simulink model "RelOrbSim"  (R2021b)
settings: Solver=ode3  StartTime=0.0  StopTime=300  FixedStep=0.1  MaxStep=0.1  RelTol=1e-13  AbsTol=1e-16
values from neighbouring files (symbols this model uses):
  cHorizon = 12    [MAIN.m]
  Controller_Engaged_flag = 1    [MAIN.m]
  CostA = 10    [MAIN.m]
  CostB = 10    [MAIN.m]
  CostRelG = 1e4    (= 10000)    [MAIN.m]
  ctrl_flag = 1    [MAIN.m]
  g0 = 9.81    [MAIN.m]
  Isp = 250    [MAIN.m]
  J2_flag = 1    [MAIN.m]
  LinSysMat = zeros(6,6)    [MAIN.m]
  M0 = M0_next    [MAIN.m]
  pHorizon = 60    [MAIN.m]
  RangeLims = [76 75.8]    [MAIN.m]
  Tmax = 0.001    [MAIN.m]
  Ts_MPC = 5    [MAIN.m]
  Y0_Chaser = Y0_Chaser_next    [MAIN.m]
  Y0_Target = Y0_Target_next    [MAIN.m]
settings Model: SimulationMode=accelerator  Creator=vvh19  LastModifiedBy=vvh19
settings SolverCC: ZeroCrossAlgorithm=Adaptive
settings DebuggingCC: IgnoredZcDiagnostic=none

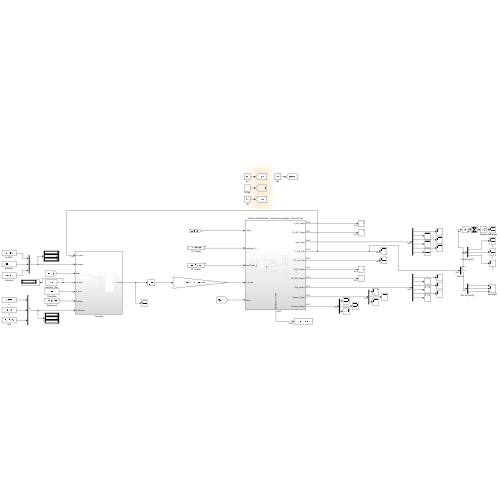
[thumbnail: Simulink's stored preview of the top-level diagram]
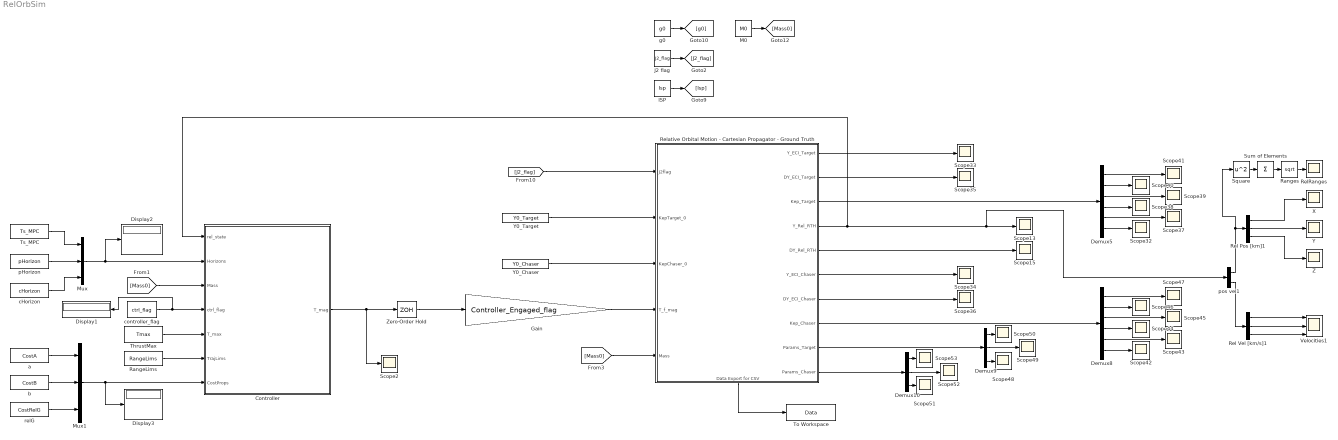
== system RelOrbSim ==
  Controller : Subsystem
  Demux10 : Demux  Outputs=3
  Demux5 : Demux  Outputs=6
  Demux8 : Demux  Outputs=6
  Demux9 : Demux  Outputs=3
  Display1 : Display
  Display2 : Display
  Display3 : Display
  Gain : Gain  Gain=Controller_Engaged_flag
  ISP : Constant  Value=Isp
  J2 flag : Constant  Value=J2_flag
  M0 : Constant  Value=M0
  Mux : Mux  Inputs=3
  Mux1 : Mux  Inputs=3
  RangeLims : Constant  Value=RangeLims
  Ranges : Sqrt  SaturateOnIntegerOverflow=on
  Rel Pos [km]1 : Demux  Outputs=3
  Rel Vel [km/s]1 : Demux  Outputs=3
  RelRanges : Scope
  Relative Orbital Motion - Cartesian Propagator - Ground Truth : Subsystem
      settings: PortSchema="{\"entries\":[{\"content\":{\"sides\":[{\"content\":{\"connectorIds\":[\"In1\",\"In2\",\"In3\",\"In4\",\"In5\"]},\"type\":\"ConnectorPlacement.EquallySpacedRectSide\",\"uuid\":\"460fd9d6-cd5d-4b76-b443-bcd8299910b0\"},{\"content\":{\"connectorIds\":[\"Out1\",\"Out2\",\"Out3\",\"Out4\",\"Out5\",\"Out6\",\"Out7\",\"Out8\",\"Out9\",\"Out10\"],\"side\":\"RIGHT\"},\"type\":\"ConnectorPlacement.EquallySpacedRectSide\",\"uuid\":\"3d6e3c75-f9f1-4d35-a2af-329ac414795a\"},{\"content\":{\"connectorIds\":[],\"side\":\"TOP\"},\"type\":\"ConnectorPlacement.EquallySpacedRectSide\",\"uuid\":\"ebced619-41c7-4fff-b50c-f89432cfa79e\"},{\"content\":{\"connectorIds\":[\"Out11\"],\"side\":\"BOTTOM\"},\"type\":\"ConnectorPlacement.EquallySpacedRectSide\",\"uuid\":\"f646bff0-d8f7-4748-8894-8aba1f3e2913\"}]},\"type\":\"ConnectorPlacement.EquallySpacedConnector\",\"uuid\":\"aa7fbb89-a653-4056-80bd-de050f54cf23\"}],\"packageUris\":[\"http://schema.mathworks.com/mf0/Connector/R2020b\"],\"version\":\"1.0\"}"
  Scope{2,13,15,32..53} (25 alike) : Scope
  Square : Math  Operator=square  SaturateOnIntegerOverflow=on
  Sum of Elements : Sum  Inputs=+
  ThrustMax : Constant  Value=Tmax
  To Workspace : ToWorkspace  VariableName=Data  SampleTime=-1
      settings: Save2DSignal=2-D array (concatenate along first dimension)
  Ts_MPC : Constant  Value=Ts_MPC
  Velocities1 : Scope  NumInputPorts=3
  X : Scope
  Y : Scope
  Y0_Chaser : Constant  Value=Y0_Chaser
  Y0_Target : Constant  Value=Y0_Target
  Z : Scope
  Zero-Order Hold : ZeroOrderHold  SampleTime=Ts_MPC
  a : Constant  Value=CostA
  b : Constant  Value=CostB
  cHorizon : Constant  Value=cHorizon
  controller_flag : Constant  Value=ctrl_flag
  g0 : Constant  Value=g0
  pHorizon : Constant  Value=pHorizon
  pos vel1 : Demux  Outputs=2
  relG : Constant  Value=CostRelG
  wires:
  ISP/1 -> [Isp]
  J2 flag/1 -> [J2_flag]
  M0/1 -> [Mass0]
  g0/1 -> [g0]
  Y0_Target/1 -> Relative Orbital Motion - Cartesian Propagator - Ground Truth/2(KepTarget_0)
  Y0_Chaser/1 -> Relative Orbital Motion - Cartesian Propagator - Ground Truth/3(KepChaser_0)
  [J2_flag] -> Relative Orbital Motion - Cartesian Propagator - Ground Truth/1(J2flag)
  Relative Orbital Motion - Cartesian Propagator - Ground Truth/4(Y_Rel_RTH) -> Scope13/1, pos vel1/1, Controller/1(rel_state)
  Relative Orbital Motion - Cartesian Propagator - Ground Truth/5(DY_Rel_RTH) -> Scope15/1
  Relative Orbital Motion - Cartesian Propagator - Ground Truth/1(Y_ECI_Target) -> Scope33/1
  Relative Orbital Motion - Cartesian Propagator - Ground Truth/6(Y_ECI_Chaser) -> Scope34/1
  Relative Orbital Motion - Cartesian Propagator - Ground Truth/2(DY_ECI_Target) -> Scope35/1
  Relative Orbital Motion - Cartesian Propagator - Ground Truth/7(DY_ECI_Chaser) -> Scope36/1
  Demux5/3 -> Scope39/1
  Demux5/2 -> Scope40/1
  Relative Orbital Motion - Cartesian Propagator - Ground Truth/3(Kep_Target) -> Demux5/1
  Demux5/4 -> Scope38/1
  Demux5/6 -> Scope32/1
  Demux5/1 -> Scope41/1
  Demux5/5 -> Scope37/1
  Demux8/5 -> Scope43/1
  Demux8/1 -> Scope47/1
  Demux8/6 -> Scope42/1
  Demux8/4 -> Scope44/1
  Relative Orbital Motion - Cartesian Propagator - Ground Truth/8(Kep_Chaser) -> Demux8/1
  Demux8/2 -> Scope46/1
  Demux8/3 -> Scope45/1
  Relative Orbital Motion - Cartesian Propagator - Ground Truth/11(Data Export for CSV) -> To Workspace/1
  Demux9/2 -> Scope49/1
  Demux9/3 -> Scope48/1
  Demux9/1 -> Scope50/1
  Relative Orbital Motion - Cartesian Propagator - Ground Truth/9(Params_Target) -> Demux9/1
  Demux10/1 -> Scope53/1
  Demux10/3 -> Scope51/1
  Demux10/2 -> Scope52/1
  Relative Orbital Motion - Cartesian Propagator - Ground Truth/10(Params_Chaser) -> Demux10/1
  pos vel1/1 -> Square/1, Rel Pos [km]1/1
  Rel Pos [km]1/1 -> X/1
  Rel Pos [km]1/3 -> Z/1
  pos vel1/2 -> Rel Vel [km/s]1/1
  Rel Pos [km]1/2 -> Y/1
  Rel Vel [km/s]1/1 -> Velocities1/1
  Rel Vel [km/s]1/2 -> Velocities1/2
  Rel Vel [km/s]1/3 -> Velocities1/3
  controller_flag/1 -> Display1/1, Controller/4(ctrl_flag)
  Square/1 -> Sum of Elements/1
  Sum of Elements/1 -> Ranges/1
  Ranges/1 -> RelRanges/1
  [Mass0] -> Controller/3(Mass)
  [Mass0] -> Relative Orbital Motion - Cartesian Propagator - Ground Truth/5(Mass)
  ThrustMax/1 -> Controller/5(T_max)
  Mux/1 -> Controller/2(Horizons), Display2/1
  pHorizon/1 -> Mux/2
  cHorizon/1 -> Mux/3
  Ts_MPC/1 -> Mux/1
  RangeLims/1 -> Controller/6(TrajLims)
  Mux1/1 -> Controller/7(CostProps), Display3/1
  a/1 -> Mux1/1
  b/1 -> Mux1/2
  Gain/1 -> Relative Orbital Motion - Cartesian Propagator - Ground Truth/4(T_f_mag)
  Controller/1(T_mag) -> Zero-Order Hold/1, Scope2/1
  Zero-Order Hold/1 -> Gain/1
  relG/1 -> Mux1/3

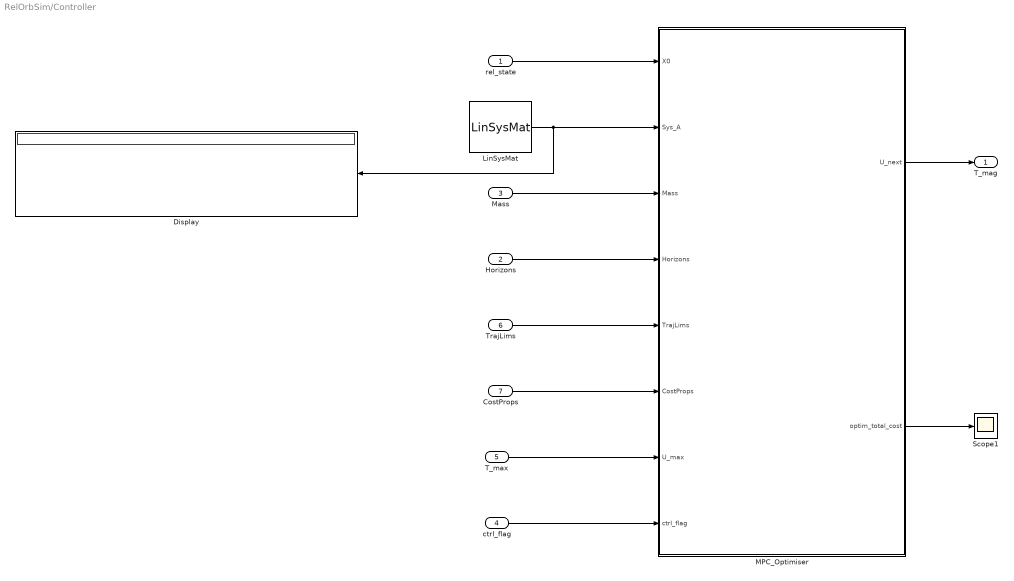
== system RelOrbSim/Controller ==
  rel_state : Inport
  Horizons : Inport  Port=2
  Mass : Inport  Port=3
  ctrl_flag : Inport  Port=4
  T_max : Inport  Port=5
  TrajLims : Inport  Port=6
  CostProps : Inport  Port=7
  Display : Display
  LinSysMat : Constant  Value=LinSysMat
  MPC_Optimiser : MATLAB Function  TreatAsAtomicUnit=on
  Scope1 : Scope
  T_mag : Outport
  wires:
  LinSysMat/1 -> Display/1, MPC_Optimiser/2(Sys_A)
  rel_state/1 -> MPC_Optimiser/1(X0)
  Mass/1 -> MPC_Optimiser/3(Mass)
  T_max/1 -> MPC_Optimiser/7(U_max)
  MPC_Optimiser/2(optim_total_cost) -> Scope1/1
  MPC_Optimiser/1(U_next) -> T_mag/1
  ctrl_flag/1 -> MPC_Optimiser/8(ctrl_flag)
  TrajLims/1 -> MPC_Optimiser/5(TrajLims)
  Horizons/1 -> MPC_Optimiser/4(Horizons)
  CostProps/1 -> MPC_Optimiser/6(CostProps)

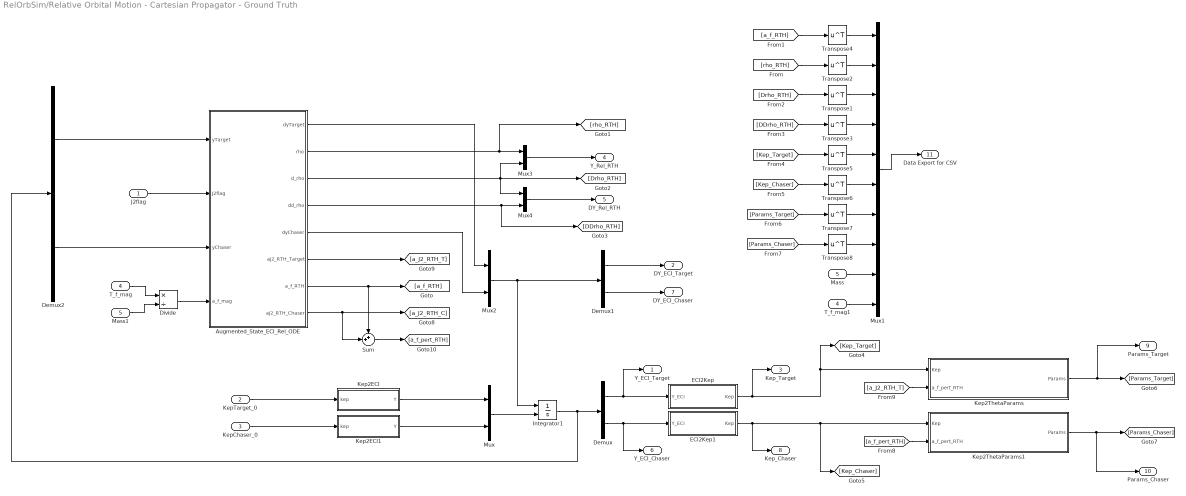
== system RelOrbSim/Relative Orbital Motion - Cartesian Propagator - Ground Truth ==
  J2flag : Inport
  KepTarget_0 : Inport  Port=2
  KepChaser_0 : Inport  Port=3
  T_f_mag : Inport  Port=4
  Mass : Inport  Port=5
  Augmented_State_ECI_Rel_ODE : MATLAB Function  TreatAsAtomicUnit=on
  Demux : Demux  Outputs=2
  Demux1 : Demux  Outputs=2
  Demux2 : Demux  Outputs=2
  Divide : Product  Inputs=*/
  ECI2Kep : MATLAB Function  TreatAsAtomicUnit=on
  ECI2Kep1 : MATLAB Function  TreatAsAtomicUnit=on
  Integrator1 : Integrator  InitialConditionSource=external  AbsoluteTolerance=1e-14
  Kep2ECI : MATLAB Function  TreatAsAtomicUnit=on
  Kep2ECI1 : MATLAB Function  TreatAsAtomicUnit=on
  Kep2ThetaParams : MATLAB Function  TreatAsAtomicUnit=on
  Kep2ThetaParams1 : MATLAB Function  TreatAsAtomicUnit=on
  Mass1 : InportShadow  Port=5
  Mux{,2..4} (4 alike) : Mux  Inputs=2
  Mux1 : Mux  Inputs=10
  Sum : Sum  Inputs=++|
  T_f_mag1 : InportShadow  Port=4
  Transpose{1..8} (8 alike) : Math  Operator=transpose  SaturateOnIntegerOverflow=on
  Y_ECI_Target : Outport
  DY_ECI_Target : Outport  Port=2
  Kep_Target : Outport  Port=3
  Y_Rel_RTH : Outport  Port=4
  DY_Rel_RTH : Outport  Port=5
  Y_ECI_Chaser : Outport  Port=6
  DY_ECI_Chaser : Outport  Port=7
  Kep_Chaser : Outport  Port=8
  Params_Target : Outport  Port=9
  Params_Chaser : Outport  Port=10
  Data Export for CSV : Outport  Port=11
  wires:
  J2flag/1 -> Augmented_State_ECI_Rel_ODE/2(J2flag)
  Mux/1 -> Integrator1/2
  KepChaser_0/1 -> Kep2ECI1/1(kep)
  KepTarget_0/1 -> Kep2ECI/1(kep)
  Kep2ECI/1(Y) -> Mux/1
  Kep2ECI1/1(Y) -> Mux/2
  Integrator1/1 -> Demux2/1, Demux/1
  Demux/1 -> ECI2Kep/1(Y_ECI), Y_ECI_Target/1
  Demux/2 -> ECI2Kep1/1(Y_ECI), Y_ECI_Chaser/1
  Mux2/1 -> Demux1/1, Integrator1/1
  Augmented_State_ECI_Rel_ODE/1(dyTarget) -> Mux2/1
  Augmented_State_ECI_Rel_ODE/5(dyChaser) -> Mux2/2
  Demux1/2 -> DY_ECI_Chaser/1
  Demux1/1 -> DY_ECI_Target/1
  Demux2/2 -> Augmented_State_ECI_Rel_ODE/3(yChaser)
  Demux2/1 -> Augmented_State_ECI_Rel_ODE/1(yTarget)
  Augmented_State_ECI_Rel_ODE/2(rho) -> [rho_RTH], Mux3/1
  Augmented_State_ECI_Rel_ODE/3(d_rho) -> Mux3/2, [Drho_RTH], Mux4/1
  Augmented_State_ECI_Rel_ODE/4(dd_rho) -> [DDrho_RTH], Mux4/2
  Mux3/1 -> Y_Rel_RTH/1
  Mux4/1 -> DY_Rel_RTH/1
  ECI2Kep/1(Kep) -> [Kep_Target], Kep2ThetaParams/1(Kep), Kep_Target/1
  ECI2Kep1/1(Kep) -> Kep2ThetaParams1/1(Kep), [Kep_Chaser], Kep_Chaser/1
  [DDrho_RTH] -> Transpose3/1
  [Drho_RTH] -> Transpose1/1
  [rho_RTH] -> Transpose2/1
  [a_f_RTH] -> Transpose4/1
  [Kep_Target] -> Transpose5/1
  [Kep_Chaser] -> Transpose6/1
  Transpose4/1 -> Mux1/1
  Transpose2/1 -> Mux1/2
  Transpose1/1 -> Mux1/3
  Transpose3/1 -> Mux1/4
  Transpose5/1 -> Mux1/5
  Transpose6/1 -> Mux1/6
  Mux1/1 -> Data Export for CSV/1
  Kep2ThetaParams/1(Params) -> [Params_Target], Params_Target/1
  Kep2ThetaParams1/1(Params) -> Params_Chaser/1, [Params_Chaser]
  [Params_Chaser] -> Transpose8/1
  [Params_Target] -> Transpose7/1
  Transpose7/1 -> Mux1/7
  Transpose8/1 -> Mux1/8
  Augmented_State_ECI_Rel_ODE/7(a_f_RTH) -> Sum/1, [a_f_RTH]
  Augmented_State_ECI_Rel_ODE/8(aJ2_RTH_Chaser) -> Sum/2, [a_J2_RTH_C]
  Augmented_State_ECI_Rel_ODE/6(aJ2_RTH_Target) -> [a_J2_RTH_T]
  Sum/1 -> [a_f_pert_RTH]
  [a_f_pert_RTH] -> Kep2ThetaParams1/2(a_f_pert_RTH)
  [a_J2_RTH_T] -> Kep2ThetaParams/2(a_f_pert_RTH)
  Mass/1 -> Mux1/9
  T_f_mag/1 -> Divide/1
  Mass1/1 -> Divide/2
  Divide/1 -> Augmented_State_ECI_Rel_ODE/4(a_f_mag)
  T_f_mag1/1 -> Mux1/10

== matlab function RelOrbSim/Relative Orbital Motion - Cartesian Propagator - Ground Truth/Kep2ThetaParams ==
  data: Params output size=3,1; Kep input; a_f_pert_RTH input
function Params = Kep2ThetaParams(Kep, a_f_pert_RTH)
%% Inputs
a = Kep(1);     e = Kep(2);     theta = Kep(6);
a_r = a_f_pert_RTH(1);      a_t = a_f_pert_RTH(2);      a_h = a_f_pert_RTH(3);

mu = 3.98600433e+5; % From DE405

r = a*(1-e^2)/(1+e*cos(theta));

kw3_2 = mu/r^3;
% dw = -2*mu*e*sin(theta) / r^3;
% w = sqrt( mu * a*(1-e^2) ) / r^2;
% 
% Params = [kw3_2; dw; w];

% Trial - Also find derivative of "w" in presence of perturbations
h = sqrt( mu * a*(1-e^2) );
p = a*(1-e^2);

w =  h / r.^2 + 1 / ( e * h ) * (p * cos( theta ) * a_r - ( p + r ) * sin( theta ) * a_t );

r_dot = e * p * w * sin( theta ) / ( 1 + e * cos( theta ) )^2;

dw = ( -2 * h * r_dot / r^3 ) + ( 1 / ( e * h ) ) *...
    ( ( w * -( a_r * p * sin(theta) + a_t * r * cos(theta) + a_t * p * cos(theta) ) )...
        - a_t * sin(theta) * r_dot );

Params = [kw3_2; dw; w];

end

== matlab function RelOrbSim/Controller/MPC_Optimiser ==
  data: X0 input; Sys_A input; Mass input; Horizons input; TrajLims input; U_next output size=[1,1]; CostProps input; U_max input; optim_total_cost output; ctrl_flag input
function [U_next, optim_total_cost] = MPC_optimiser(X0, Sys_A, Mass, Horizons, TrajLims, CostProps, U_max, ctrl_flag)

% *********************************************************************** %
Sys_A = Sys_A*1e-3*1e3; % Confirm This - Python is in [m], Matlab is in [km]
% *********************************************************************** %

if ctrl_flag == 0
    U_next = 0;     optim_total_cost = 0;
else
    Guess_TP = [0, 0];
    
    optim_opts = optimoptions("fmincon", "Algorithm",'sqp',...
                              "ConstraintTolerance", 1e-6,...
                              "MaxIterations", 50, ...
                              "ScaleProblem",true);
    
    [optim_profile, optim_total_cost] = fmincon(@(TP)...
        MPCobjective(TP, X0, Sys_A, Mass, Horizons, TrajLims, CostProps),...
        Guess_TP,...
        [], [], ...
        [], [], ...
        [-U_max, 0], [U_max, 5], ...
        [], ...
        optim_opts);
    
    Ta = optim_profile(1);
    Tb = optim_profile(2);
    
    Ts = Horizons(1);
    U_next = (Ta*exp(-Tb*Ts));
    U_next = Ta;
end

end

%%%%%%%%%%%%%%%%%%%%%%%%%%%%%%%%%%%%%%%%%%%%%%%%%%%%%%%%%%%%%%%%%%%%%%%%%%%

function TotalCost = MPCobjective(TP, X0, Sys_A, Mass, Horizons, TrajLims, CostProps)
% Objective function for MPC optimisation Loop

%% Initialisation
a = TP(1);      b = TP(2);
Sys_B = [zeros(3,3); eye(3)./Mass];

% Horizons
Ts = Horizons(1);       pH = Horizons(2);       cH = Horizons(3);

% Traj Limits
M_rng = TrajLims(1); % max range bounds [km]
m_rng = TrajLims(2); % min range bounds [km]

% Cost
a_cost = CostProps(1); % Amplitude factor for Area under minimum violation cost
b_cost = CostProps(2); %  Amplitude factor/ slope for maximum violation cost
CtrlCost_Gain = CostProps(3);

%% Thrust Profile
U = @(t) (a*exp(-b*t)).*(t<=Ts*cH);
thrust_pointing = @(X) -X(1:3)./norm(X(1:3));

%% Propagation
X_dot = @(t, X) Sys_A*X + Sys_B*thrust_pointing(X)*U(t);
tspan = 0:Ts:Ts*pH;
ode_opt = odeset('RelTol',1e-5,'AbsTol',1e-6);
[~,y] = ode45(@(t, X) X_dot(t, X), tspan, X0, ode_opt);

%% Cost Calculations
ranges = vecnorm(y(:,1:3)'); % [km]

costFn = @(ranges) (m_rng - min(m_rng, ranges))*a_cost + (max(M_rng, ranges) - M_rng)*b_cost;

TrajCost = sum(costFn(ranges))/length(ranges);
CtrlCost = sum(abs(U(tspan)))*CtrlCost_Gain/(Ts*cH);
TotalCost = TrajCost + CtrlCost;

end

== matlab function RelOrbSim/Relative Orbital Motion - Cartesian Propagator - Ground Truth/Augmented_State_ECI_Rel_ODE ==
  data: dyTarget output size=6,1; rho output size=3,1; d_rho output size=3,1; dd_rho output size=3,1; yTarget input; J2flag input; yChaser input; dyChaser output size=6,1; aJ2_RTH_Target output size=3,1; a_f_mag input; a_f_RTH output size=3,1; aJ2_RTH_Chaser output size=3,1
function [dyTarget, rho, d_rho, dd_rho, dyChaser, aJ2_RTH_Target, a_f_RTH, aJ2_RTH_Chaser] = ode_2BP_Earth(yTarget, J2flag, yChaser, a_f_mag)

mu = 3.98600433e+5; % From DE405
R_E = 6378.1363; % use for J2 only [km] 

if J2flag == 0
    J2 = 0;
else  
    J2 = 0.1082626925638815e-2; % J2 value (Definition in Wertz, SMAD)
end

% Relative RTH State Vector
r_T = yTarget(1:3);    v_T = yTarget(4:6);     
r_C = yChaser(1:3);    v_C = yChaser(4:6);      

% Construct Target Centered RTH Frame
x_cap = r_T./norm(r_T);
z_cap = ( cross(r_T, v_T) ./ norm(cross(r_T, v_T)) );
y_cap = cross(z_cap, x_cap) ./ norm(cross(z_cap, x_cap));
T = [x_cap, y_cap, z_cap]';

rho_ECI = r_C - r_T;    rho_dot_ECI = v_C - v_T;    

% Control Accelerations
rho_cap_ECI = rho_ECI./norm(rho_ECI);
thrust_cap_ECI = -rho_cap_ECI;
a_f_ECI = thrust_cap_ECI*a_f_mag;

% Outputs - 1
[dyTarget, aJ2_vect_ECEI_Target] = ode_2BP_perturbed_J2(yTarget, mu, R_E, J2, [0;0;0] );
[dyChaser, aJ2_vect_ECEI_Chaser] = ode_2BP_perturbed_J2(yChaser, mu, R_E, J2, a_f_ECI );

dv_T = dyTarget(4:6);      dv_C = dyChaser(4:6);       rho_dotdot_ECI = dv_C - dv_T;

% Outputs - 2
rho = T*rho_ECI;        d_rho = T*rho_dot_ECI;    dd_rho =  T*rho_dotdot_ECI;
aJ2_RTH_Target = T*aJ2_vect_ECEI_Target;    aJ2_RTH_Chaser = T*aJ2_vect_ECEI_Chaser;

rho_cap_RTH = rho./norm(rho);
thrust_cap_RTH = -rho_cap_RTH; 
a_f_RTH = thrust_cap_RTH*a_f_mag;

end

%%%%%%%%%%%%%%%%%%%%%%%%%%%%%%%%%%%%%%%%%%%%%%%%%%%%%%%%%%%%%%%%%%%%%%%%%%%

function [dy, aJ2_vect_ECEI] = ode_2BP_perturbed_J2(y, mu, R_E, J2, a_f_ECI )
r = y(1:3);
r_norm = norm(r);
v = y(4:6);

aJ2_vect_ECEI = 3/2 * J2 * mu * R_E^2 / r_norm^5 *       ... % Multiplicative constant
    [ r(1) * ( 5 * (r(3) / r_norm)^2 - 1 );   ... % x-component
      r(2) * ( 5 * (r(3) / r_norm)^2 - 1 );   ... % y-component
      r(3) * ( 5 * (r(3) / r_norm)^2 - 3 )];      % z-component

dy = [ v; -mu ./ r_norm.^3 .* r + aJ2_vect_ECEI + a_f_ECI];

end

== matlab function RelOrbSim/Relative Orbital Motion - Cartesian Propagator - Ground Truth/Kep2ECI ==
  data: Y output; kep input
function Y = Kep2Car( kep )
%% Inputs
a = kep(1);     e = kep(2);     i = kep(3);
OM = kep(4);    om = kep(5);    theta = kep(6);
mu = 3.98600433e+5; % From DE405

%% Calculate r, v in perifocal frame
unit_r = [cos(theta); sin(theta); 0];
unit_theta = [-sin(theta); cos(theta); 0];
P = a.*(1-e.^2);

r_pf = a .* (1 - e.^2) ./ (1 + e .* cos(theta)) * unit_r; % r in perifocal plane
v_r = sqrt( mu ./ P ) .* e .* sin(theta) * unit_r;
v_theta = sqrt( mu ./ P ) .* ( 1 + e .* cos(theta) ) * unit_theta;

v_pf = v_r + v_theta;

%% Calculate rotation matrix

R_OM  = [  cos(OM), sin(OM), 0       ;
          -sin(OM), cos(OM), 0       ;
           0,       0,       1      ];

R_i  = [   1,       0,       0       ;
           0,       cos(i),  sin(i)  ;
           0,      -sin(i),  cos(i) ];

R_om = [   cos(om), sin(om), 0                     
          -sin(om), cos(om), 0
           0,       0,       1,     ];

R_ECEI2PF = R_om*R_i*R_OM;

r = R_ECEI2PF'*r_pf;
v = R_ECEI2PF'*v_pf;

%% Generate State Vector
Y = [r;v];
end

== matlab function RelOrbSim/Relative Orbital Motion - Cartesian Propagator - Ground Truth/Kep2ThetaParams1 ==
  data: Params output size=3,1; Kep input; a_f_pert_RTH input
function Params = Kep2ThetaParams(Kep, a_f_pert_RTH)
%% Inputs
a = Kep(1);     e = Kep(2);     theta = Kep(6);
a_r = a_f_pert_RTH(1);      a_t = a_f_pert_RTH(2);      a_h = a_f_pert_RTH(3);

mu = 3.98600433e+5; % From DE405

r = a*(1-e^2)/(1+e*cos(theta));

kw3_2 = mu/r^3;
% dw = -2*mu*e*sin(theta) / r^3;
% w = sqrt( mu * a*(1-e^2) ) / r^2;
% 
% Params = [kw3_2; dw; w];

% Trial - Also find derivative of "w" in presence of perturbations
h = sqrt( mu * a*(1-e^2) );
p = a*(1-e^2);

w =  h / r.^2 + 1 / ( e * h ) * (p * cos( theta ) * a_r - ( p + r ) * sin( theta ) * a_t );

r_dot = e * p * w * sin( theta ) / ( 1 + e * cos( theta ) )^2;

dw = ( -2 * h * r_dot / r^3 ) + ( 1 / ( e * h ) ) *...
    ( ( w * -( a_r * p * sin(theta) + a_t * r * cos(theta) + a_t * p * cos(theta) ) )...
        - a_t * sin(theta) * r_dot );

Params = [kw3_2; dw; w];

end

== matlab function RelOrbSim/Relative Orbital Motion - Cartesian Propagator - Ground Truth/Kep2ECI1 ==
  data: Y output; kep input
function Y = Kep2Car( kep )
%% Inputs
a = kep(1);     e = kep(2);     i = kep(3);
OM = kep(4);    om = kep(5);    theta = kep(6);
mu = 3.98600433e+5; % From DE405

%% Calculate r, v in perifocal frame
unit_r = [cos(theta); sin(theta); 0];
unit_theta = [-sin(theta); cos(theta); 0];
P = a.*(1-e.^2);

r_pf = a .* (1 - e.^2) ./ (1 + e .* cos(theta)) * unit_r; % r in perifocal plane
v_r = sqrt( mu ./ P ) .* e .* sin(theta) * unit_r;
v_theta = sqrt( mu ./ P ) .* ( 1 + e .* cos(theta) ) * unit_theta;

v_pf = v_r + v_theta;

%% Calculate rotation matrix

R_OM  = [  cos(OM), sin(OM), 0       ;
          -sin(OM), cos(OM), 0       ;
           0,       0,       1      ];

R_i  = [   1,       0,       0       ;
           0,       cos(i),  sin(i)  ;
           0,      -sin(i),  cos(i) ];

R_om = [   cos(om), sin(om), 0                     
          -sin(om), cos(om), 0
           0,       0,       1,     ];

R_ECEI2PF = R_om*R_i*R_OM;

r = R_ECEI2PF'*r_pf;
v = R_ECEI2PF'*v_pf;

%% Generate State Vector
Y = [r;v];
end

== matlab function RelOrbSim/Relative Orbital Motion - Cartesian Propagator - Ground Truth/ECI2Kep ==
  data: Kep output size=6,1; Y_ECI input
function Kep = Car2Kep(Y_ECI)
% Calculate parameters
r_ECI = Y_ECI(1:3);
v_ECI = Y_ECI(4:6);
mu = 3.98600433e+5; % From DE405

% This tolerance is required to have accurate results from MATLAB
tol = .2e-15;

% Define xyz axis
x = [ 1, 0, 0 ];
y = [ 0, 1, 0 ];
z = [ 0, 0, 1 ];

r_norm = norm(r_ECI);

% Calculate semi-major axis
a = 1 ./ ( 2 ./ r_norm - norm(v_ECI).^2 ./ mu );

% Calculate angular momentum vector
h_ECI = cross( r_ECI, v_ECI );

% Calculate eccentricity vector
e = cross( v_ECI, h_ECI ) ./ mu - r_ECI ./ r_norm;
e_norm = norm(e);

% Calculate inclination
i = acos( dot( h_ECI, z ) ./ norm(h_ECI) ); % 0<i<pi
%%%%%%%%%%%%%%%%%%%%%%%%%%%%%%%%%%%%%%%%%%%%%%%%%%%%%%%%%%%%%%%%%%%%%%%%%%%
if i - tol < 0
    % RAAN is undefined if i = 0 ( i < tol )
    OM = 0;
    AN = [1;0;0];
else
    % RAAN is defined
    % Calculate ascending node (AN)
    AN = cross( z, h_ECI ) ./ norm( cross( z, h_ECI ) ); % Ascending node unit vector
    % Solve OM angle ambiguity
    if dot( AN, y ) > 0 % 0<OM<2pi
        OM = acos( dot( x, AN ) );
    elseif dot( AN, y ) < 0 % 0<OM<2pi
        OM = 2*pi - acos( dot( x, AN ) );
    else % dot( AN, y ) = 0
        % In this case, OM could be 0 or 180 ???? -> Check if it can
        % actually be 180 because idk
        OM = 0;
    end
end

if e_norm - tol > 0
    % om is defined
    % Solve om angular ambiguity
    if dot( z, e ) >= 0
        om = acos( dot(AN, e) ./ e_norm );
    elseif dot( z, e ) < 0
        om = 2*pi - acos( dot(AN, e) ./ e_norm );
    else
        om = 0;
    end
else
    % om is undefined if e = 0 ( e < tol )
    om = 0;
end

if e_norm - tol > 0
    % theta can be calculated from eccentricity vector if e_norm > tol
    % Solve theta angular ambiguity
    K = dot( r_ECI, e ) ./ ( r_norm .* e_norm );
    k = max(min(K,1),-1);
    if dot( r_ECI, v_ECI ) >= 0
        theta = acos( k );
    elseif dot( r_ECI, v_ECI ) < 0
        theta = 2*pi - acos( k );
    else
        theta = 0;
    end
else
    % theta cannot be calculated from eccentricity vector if e_norm < tol
    % Set theta to start from x-axis and solve for angular ambiguity
    if dot( r_ECI, v_ECI ) >= 0
        theta = acos( dot( r_ECI, x ) ./ ( r_norm ) );
    elseif dot( r_ECI, v_ECI ) < 0
        theta = 2*pi - acos( dot( r_ECI, x ) ./ ( r_norm ) );
    else
        theta = 0;
    end
    % If you arrive in this if, e_norm < tol -> it was actually 0
    e_norm = 0;
end
%%%%%%%%%%%%%%%%%%%%%%%%%%%%%%%%%%%%%%%%%%%%%%%%%%%%%%%%%%%%%%%%%%%%%%%%%%%
om = om(1);
Kep = zeros(6,1);
Kep = [ a, e_norm, i, OM, om, theta ]';
end

== matlab function RelOrbSim/Relative Orbital Motion - Cartesian Propagator - Ground Truth/ECI2Kep1 ==
  data: Kep output size=6,1; Y_ECI input
function Kep = Car2Kep(Y_ECI)
% Calculate parameters
r_ECI = Y_ECI(1:3);
v_ECI = Y_ECI(4:6);
mu = 3.98600433e+5; % From DE405

% This tolerance is required to have accurate results from MATLAB
tol = .2e-15;

% Define xyz axis
x = [ 1, 0, 0 ];
y = [ 0, 1, 0 ];
z = [ 0, 0, 1 ];

r_norm = norm(r_ECI);

% Calculate semi-major axis
a = 1 ./ ( 2 ./ r_norm - norm(v_ECI).^2 ./ mu );

% Calculate angular momentum vector
h_ECI = cross( r_ECI, v_ECI );

% Calculate eccentricity vector
e = cross( v_ECI, h_ECI ) ./ mu - r_ECI ./ r_norm;
e_norm = norm(e);

% Calculate inclination
i = acos( dot( h_ECI, z ) ./ norm(h_ECI) ); % 0<i<pi
%%%%%%%%%%%%%%%%%%%%%%%%%%%%%%%%%%%%%%%%%%%%%%%%%%%%%%%%%%%%%%%%%%%%%%%%%%%
if i - tol < 0
    % RAAN is undefined if i = 0 ( i < tol )
    OM = 0;
    AN = [1;0;0];
else
    % RAAN is defined
    % Calculate ascending node (AN)
    AN = cross( z, h_ECI ) ./ norm( cross( z, h_ECI ) ); % Ascending node unit vector
    % Solve OM angle ambiguity
    if dot( AN, y ) > 0 % 0<OM<2pi
        OM = acos( dot( x, AN ) );
    elseif dot( AN, y ) < 0 % 0<OM<2pi
        OM = 2*pi - acos( dot( x, AN ) );
    else % dot( AN, y ) = 0
        % In this case, OM could be 0 or 180 ???? -> Check if it can
        % actually be 180 because idk
        OM = 0;
    end
end

if e_norm - tol > 0
    % om is defined
    % Solve om angular ambiguity
    if dot( z, e ) >= 0
        om = acos( dot(AN, e) ./ e_norm );
    elseif dot( z, e ) < 0
        om = 2*pi - acos( dot(AN, e) ./ e_norm );
    else
        om = 0;
    end
else
    % om is undefined if e = 0 ( e < tol )
    om = 0;
end

if e_norm - tol > 0
    % theta can be calculated from eccentricity vector if e_norm > tol
    % Solve theta angular ambiguity
    K = dot( r_ECI, e ) ./ ( r_norm .* e_norm );
    k = max(min(K,1),-1);
    if dot( r_ECI, v_ECI ) >= 0
        theta = acos( k );
    elseif dot( r_ECI, v_ECI ) < 0
        theta = 2*pi - acos( k );
    else
        theta = 0;
    end
else
    % theta cannot be calculated from eccentricity vector if e_norm < tol
    % Set theta to start from x-axis and solve for angular ambiguity
    if dot( r_ECI, v_ECI ) >= 0
        theta = acos( dot( r_ECI, x ) ./ ( r_norm ) );
    elseif dot( r_ECI, v_ECI ) < 0
        theta = 2*pi - acos( dot( r_ECI, x ) ./ ( r_norm ) );
    else
        theta = 0;
    end
    % If you arrive in this if, e_norm < tol -> it was actually 0
    e_norm = 0;
end
%%%%%%%%%%%%%%%%%%%%%%%%%%%%%%%%%%%%%%%%%%%%%%%%%%%%%%%%%%%%%%%%%%%%%%%%%%%
om = om(1);
Kep = zeros(6,1);
Kep = [ a, e_norm, i, OM, om, theta ]';
end
